simulink model "Demo_fin"  (R2022b)
settings: Solver=ode23tb  StartTime=0.0  StopTime=630  FixedStep=0.001  RelTol=1e-2
settings Model: Creator=Maxim Kozlov  LastModifiedBy=KozlovM
settings OptimizationCC: ReuseModelBlockBuffer=on
settings ModelReferenceCC: EnableParallelModelReferenceBuilds=on  UseModelRefSolver=on

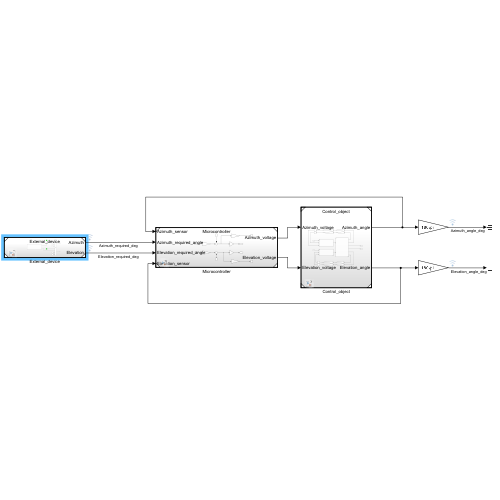
[thumbnail: Simulink's stored preview of the top-level diagram]
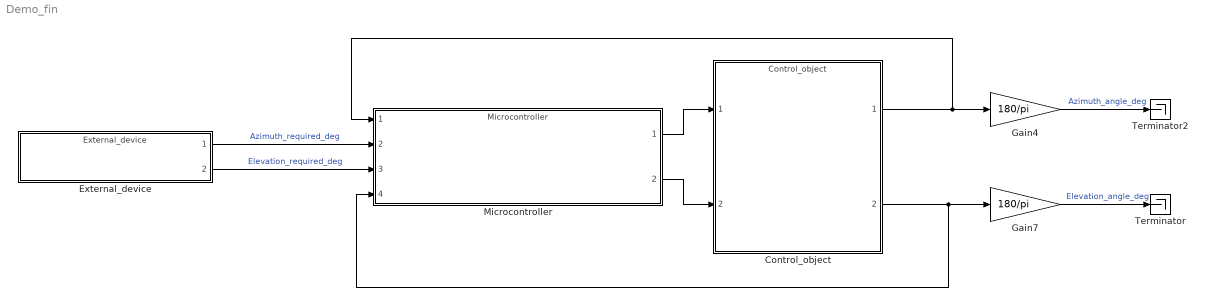
== system Demo_fin ==
  Control_object : ModelReference  ModelNameDialog=Control_object.slx  SimulationMode=Normal  ModelReferenceVersion=2.5  InputSignalHandling=Zero-order hold
  External_device : ModelReference  ModelNameDialog=External_device.slx  SimulationMode=Normal  ModelReferenceVersion=1.4
  Gain4 : Gain  Gain=180/pi
  Gain7 : Gain  Gain=180/pi
  Microcontroller : ModelReference  ModelNameDialog=Microcontroller.slx  SimulationMode=Normal  ModelReferenceVersion=2.1  InputSignalHandling=Zero-order hold
  Terminator : Terminator
  Terminator2 : Terminator
  wires:
  Control_object/2 -> Gain7/1, Microcontroller/4
  External_device/2 -> Microcontroller/3  "Elevation_required_deg"
  Gain7/1 -> Terminator/1  "Elevation_angle_deg"
  Control_object/1 -> Gain4/1, Microcontroller/1
  Microcontroller/2 -> Control_object/2
  External_device/1 -> Microcontroller/2  "Azimuth_required_deg"
  Gain4/1 -> Terminator2/1  "Azimuth_angle_deg"
  Microcontroller/1 -> Control_object/1
